simulink model "PHASE3_INVERTER_RLOAD"  (R2021a)
settings: Solver=VariableStepAuto  StartTime=0.0  StopTime=10.0  RelTol=1e-3
libraries: spsMosfetLib x6, simulink x3, spsSeriesRLCBranchLib x3, spsVoltageMeasurementLib x2, spsDCVoltageSourceLib x1, spsCurrentMeasurementLib x1, spsSawtoothGeneratorLib x1, spspowerguiLib x1
settings Model: Creator=vishw  LastModifiedBy=vishw

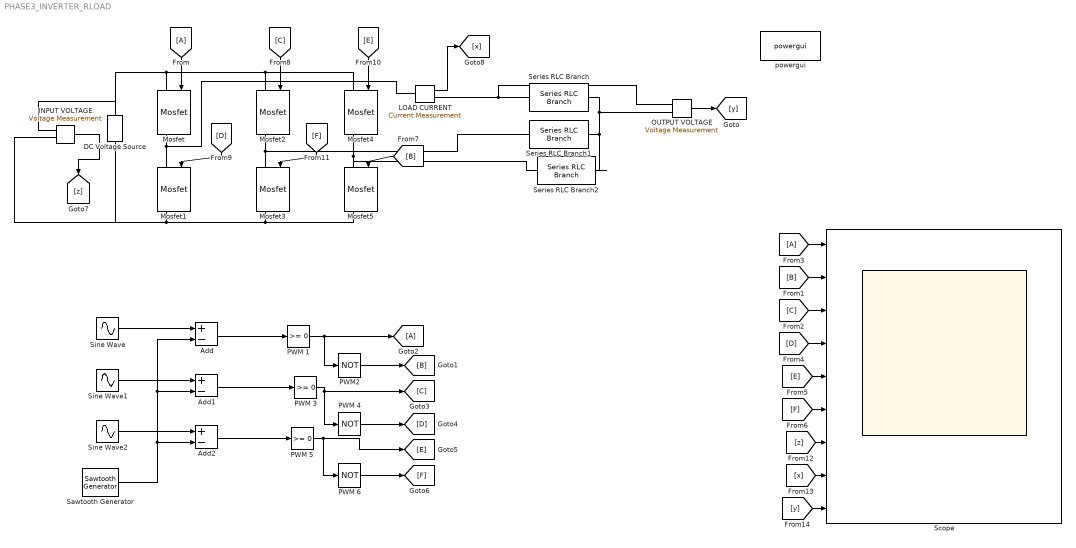
== system PHASE3_INVERTER_RLOAD ==
  Add : Sum  Inputs=+-
  Add1 : Sum  Inputs=+-
  Add2 : Sum  Inputs=+-
  DC Voltage Source : spsDCVoltageSourceLib/DC Voltage Source  Amplitude=5  Measurements=None
  INPUT VOLTAGE : spsVoltageMeasurementLib/Voltage Measurement  PhasorSimulation=off  OutputType=Complex  PSBequivalent=0
  LOAD CURRENT : spsCurrentMeasurementLib/Current Measurement  PhasorSimulation=off  OutputType=Complex  PSBequivalent=0
  Mosfet{,1..5} (6 alike) : spsMosfetLib/Mosfet  Ron=0.1  Lon=0  Rd=0.01  Vfd=0  IC=0  Rs=1e5  Cs=inf  Measurements=on
  OUTPUT VOLTAGE : spsVoltageMeasurementLib/Voltage Measurement  PhasorSimulation=off  OutputType=Complex  PSBequivalent=0
  PWM 1 : simulink/Logic and Bit Operations/Compare To Zero  relop=>=  OutDataTypeStr=boolean
  PWM 3 : simulink/Logic and Bit Operations/Compare To Zero  relop=>=  OutDataTypeStr=boolean
  PWM 4 : Logic  Operator=NOT  Inputs=1  AllPortsSameDT=off  OutDataTypeStr=boolean
  PWM 5 : simulink/Logic and Bit Operations/Compare To Zero  relop=>=  OutDataTypeStr=boolean
  PWM 6 : Logic  Operator=NOT  Inputs=1  AllPortsSameDT=off  OutDataTypeStr=boolean
  PWM2 : Logic  Operator=NOT  Inputs=1  AllPortsSameDT=off  OutDataTypeStr=boolean
  Sawtooth Generator : spsSawtoothGeneratorLib/Sawtooth Generator  Freq=1e3  Phase=180  Ts=0
  Scope : Scope  NumInputPorts=9
  Series RLC Branch : spsSeriesRLCBranchLib/Series RLC Branch  LConnTagsString=__new0  RConnTagsString=__new0  BranchType=R  Resistance=10  Inductance=1e-3  SetiL0=off  InitialCurrent=0  Capacitance=1e-6  Setx0=off  InitialVoltage=0  Measurements=None
  Series RLC Branch1 : spsSeriesRLCBranchLib/Series RLC Branch  LConnTagsString=__new0  RConnTagsString=__new0  BranchType=R  Resistance=10  Inductance=1e-3  SetiL0=off  InitialCurrent=0  Capacitance=1e-6  Setx0=off  InitialVoltage=0  Measurements=None
  Series RLC Branch2 : spsSeriesRLCBranchLib/Series RLC Branch  LConnTagsString=__new0  RConnTagsString=__new0  BranchType=R  Resistance=10  Inductance=1e-3  SetiL0=off  InitialCurrent=0  Capacitance=1e-6  Setx0=off  InitialVoltage=0  Measurements=None
  Sine Wave : Sin  Frequency=2*pi*50  SampleTime=0
  Sine Wave1 : Sin  Frequency=2*pi*50  Phase=2*pi/3  SampleTime=0
  Sine Wave2 : Sin  Frequency=2*pi*50  Phase=-2*pi/3  SampleTime=0
  powergui : spspowerguiLib/powergui  Priority=1  SimulationMode=Continuous  SampleTime=50e-6  frequency=60  Iterations=50  frequencyindice=0  Pbase=100e6  ErrMax=1e-4  UnitsV=kV  UnitsW=MW  buscounter=0  FunctionMessages=off  echomessages=off  EnableUseOfTLC=off  CurrentSourceSwitches=off  DisableSnubberDevices=off  DisableRonSwitches=off  DisableVfSwitches=off  DisplayEquations=off  AutomaticDiscreteSolvers=off  SolverType=Tustin/Backward Euler (TBE)  Interpol=off  ExternalGateDelay=off  methode=off  Ts=100  x0status=blocks  SPID=on  SwTol=0  HookPort=off  NonlinearTolerance=1e-4  nMaxIteration=100  ContinueOnMaxIteration=off  RestoreLinks=warning  ResistiveCurrentMeasurement=off  Frange=[0:2:500]  Ylog=off  Xlog=on  ShowGrid=off  save=off  variable=ZData  structure=0  ZoomFFT=off  StartTime=0.0  cycles=1  DisplayStyle=1  fundamental=60  FreqAxis=off  MaxFrequency=1000  frequencyindicesteady=1  RmsSteady=1  display=off
  wires:
  Sawtooth Generator/1 -> Add2/2, Add1/2, Add/2
  PWM 1/1 -> PWM2/1, [A]
  Sine Wave/1 -> Add/1
  Sine Wave1/1 -> Add1/1
  PWM 5/1 -> PWM 6/1, [E]
  PWM2/1 -> [B]
  Add/1 -> PWM 1/1
  PWM 6/1 -> [F]
  PWM 4/1 -> [D]
  Add1/1 -> PWM 3/1
  Sine Wave2/1 -> Add2/1
  Add2/1 -> PWM 5/1
  PWM 3/1 -> [C], PWM 4/1
  [D] -> Mosfet1/1
  [F] -> Mosfet3/1
  [B] -> Mosfet5/1
  [E] -> Mosfet4/1
  [C] -> Mosfet2/1
  [A] -> Mosfet/1
  [F] -> Scope/6
  [A] -> Scope/1
  [E] -> Scope/5
  [C] -> Scope/3
  [B] -> Scope/2
  [D] -> Scope/4
  LOAD CURRENT/1 -> [x]
  OUTPUT VOLTAGE/1 -> [y]
  INPUT VOLTAGE/1 -> [z]
  [z] -> Scope/7
  [x] -> Scope/8
  [y] -> Scope/9
  connections:
  Series RLC Branch/LConn1 -- LOAD CURRENT/RConn1 -- OUTPUT VOLTAGE/LConn1
  Mosfet3/LConn1 -- Series RLC Branch1/LConn1 -- Mosfet2/RConn1
  Mosfet5/LConn1 -- Series RLC Branch2/LConn1 -- Mosfet4/RConn1
  Mosfet5/RConn1 -- DC Voltage Source/LConn1 -- INPUT VOLTAGE/LConn2 -- Mosfet1/RConn1 -- Mosfet3/RConn1
  Mosfet/LConn1 -- INPUT VOLTAGE/LConn1 -- DC Voltage Source/RConn1 -- Mosfet4/LConn1 -- Mosfet2/LConn1
  Series RLC Branch/RConn1 -- OUTPUT VOLTAGE/LConn2 -- Series RLC Branch2/RConn1 -- Series RLC Branch1/RConn1
  Mosfet1/LConn1 -- LOAD CURRENT/LConn1 -- Mosfet/RConn1
